simulink model "facedetection_demp"  (R2021b)
settings: Solver=FixedStepAuto  StartTime=0.0  StopTime=inf  RelTol=1e-3
undefined symbols (not defined in the file): Rec, SDTV
libraries: androiduilib x5, visionconversions x3, androidaudiovideolib x2, visiontextngfix x2, androidcommunicationlib x1
settings Model: Creator=The MathWorks, Inc.  LastModifiedBy=86150
settings SolverCC: AlgebraicLoopSolver=TrustRegion
settings DataIOCC: ReturnWorkspaceOutputs=off
settings OptimizationCC: EnhancedBackFolding=on  PassReuseOutputArgsThreshold=0  MaxStackSize=64  OptimizeBlockOrder=speed  DifferentSizesBufferReuse=on  OptimizationCustomize=off
settings DebuggingCC: ParameterTunabilityLossMsg=error  SFMachineParentedDataDiag=warning  ArithmeticOperatorsInVariantConditions=warning
settings HardwareCC: ProdBitPerPointer=32  ProdBitPerSizeT=32  ProdBitPerPtrDiffT=32  ProdLargestAtomicInteger=Long  ProdLargestAtomicFloat=Double  ProdWordSize=32  ProdHWDeviceType=ARM Compatible->ARM Cortex  UseEmbeddedCoderFeatures=off  UseSimulinkCoderFeatures=off
settings SFSimCC: CustomCodeUndefinedFunction=UseInterfaceOnly
settings RTWCC: Description=Embedded Coder  SystemTargetFile=ert.tlc  HardwareBoard=Android Device  TLCOptions="-aInlineSetEventsForThisBaseRateFcn=TLC_FALSE -aSuppressMultiTaskScheduler=TLC_FALSE  -aRateBasedStepFcn=0"  TemplateMakefile=ert_default_tmf  GenerateReport=on  RTWVerbose=off  Toolchain=Android SDK/NDK Tools  LaunchReport=on
settings CodeAppCC: ForceParamTrailComments=on  OperatorAnnotations=on
settings ERTTargetCC: ERTCustomFileBanners=off  SupportContinuousTime=on  SupportNonInlinedSFcns=on  RemoveResetFunc=off  SupportVariableSizeSignals=on  ModelStepFunctionPrototypeControlCompliant=off

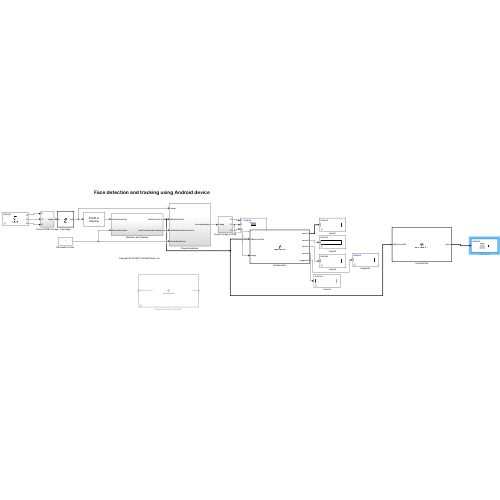
[thumbnail: Simulink's stored preview of the top-level diagram]
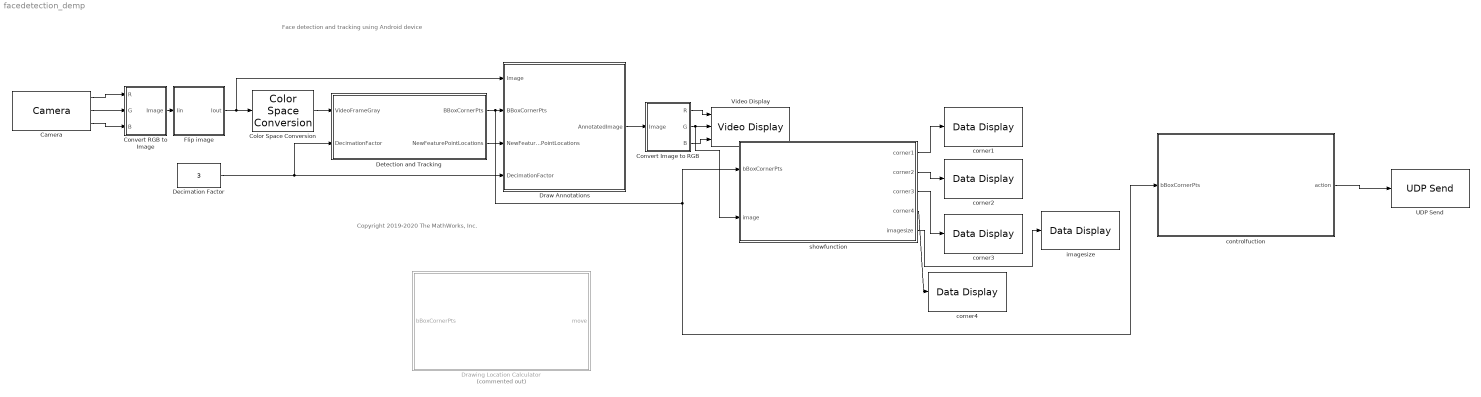
== system facedetection_demp ==
  note: Face detection and tracking using Android device
  note: Copyright 2019-2020 The MathWorks, Inc.
  Camera : androidaudiovideolib/Camera  CameraLocation=Back  CameraResolutions=Back - 640x480  Width=640  Height=480  SampleTime=0.1  BlockPlatform=Android
      settings: SourceProductBaseCode=ANDROID
  Color Space Conversion : visionconversions/Color Space  Conversion  conversion=Obsolete  conversionActive=R'G'B' to intensity  wp_str=D65  rec=Rec. 601 (SDTV)  sys=1125/60/2:1  imagePorts=One multidimensional signal
  Convert Image to RGB : Subsystem
  Convert RGB to Image : Subsystem
  Decimation Factor : Constant  Value=3
  Detection and Tracking : Subsystem
  Draw Annotations : Subsystem
  Drawing Location Calculator : MATLAB Function  Commented=on  TreatAsAtomicUnit=on
  Flip image : MATLAB Function  TreatAsAtomicUnit=on
  UDP Send : androidcommunicationlib/UDP Send  remoteURL='192.168.1.109'  remotePort=25000  localURL='0.0.0.0'  localPortSource=Automatically determine  localPort=-1  sampletime=-1  blockPlatform=Android  separateLengthPort=0
      settings: SourceProductBaseCode=ANDROID
  Video Display : androidaudiovideolib/Video Display  BlockPlatform=Android
      settings: SourceProductBaseCode=ANDROID
  controlfuction : MATLAB Function  TreatAsAtomicUnit=on
  corner1 : androiduilib/Data Display  DataDisplayId=facedetection_demp/corner1  Format=Float  Precision=6  SimulateUsing=Code generation  blockPlatform=Android
      settings: SourceProductBaseCode=ANDROID
  corner2 : androiduilib/Data Display  DataDisplayId=facedetection_demp/corner2  Format=Float  Precision=6  SimulateUsing=Code generation  blockPlatform=Android
      settings: SourceProductBaseCode=ANDROID
  corner3 : androiduilib/Data Display  DataDisplayId=facedetection_demp/corner3  Format=Float  Precision=6  SimulateUsing=Code generation  blockPlatform=Android
      settings: SourceProductBaseCode=ANDROID
  corner4 : androiduilib/Data Display  DataDisplayId=facedetection_demp/corner4  Format=Float  Precision=6  SimulateUsing=Code generation  blockPlatform=Android
      settings: SourceProductBaseCode=ANDROID
  imagesize : androiduilib/Data Display  DataDisplayId=facedetection_demp/imagesize  Format=Float  Precision=6  SimulateUsing=Code generation  blockPlatform=Android
      settings: SourceProductBaseCode=ANDROID
  showfunction : MATLAB Function  TreatAsAtomicUnit=on
  wires:
  Detection and Tracking/2(NewFeaturePointLocations) -> Draw Annotations/3(NewFeaturePointLocations)
  Detection and Tracking/1(BBoxCornerPts) -> controlfuction/1(bBoxCornerPts), showfunction/1(bBoxCornerPts), Draw Annotations/2(BBoxCornerPts)
  Color Space Conversion/1 -> Detection and Tracking/1(VideoFrameGray)
  Flip image/1(Iout) -> Draw Annotations/1(Image), Color Space Conversion/1
  Draw Annotations/1(AnnotatedImage) -> Convert Image to RGB/1(Image)
  Convert Image to RGB/1(R) -> Video Display/1
  Convert Image to RGB/2(G) -> showfunction/2(image), Video Display/2
  Convert Image to RGB/3(B) -> Video Display/3
  Convert RGB to Image/1(Image) -> Flip image/1(Iin)
  Camera/1 -> Convert RGB to Image/1(R)
  Camera/2 -> Convert RGB to Image/2(G)
  Camera/3 -> Convert RGB to Image/3(B)
  Decimation Factor/1 -> Draw Annotations/4(DecimationFactor), Detection and Tracking/2(DecimationFactor)
  showfunction/1(corner1) -> corner1/1
  showfunction/4(corner4) -> corner4/1
  showfunction/3(corner3) -> corner3/1
  showfunction/2(corner2) -> corner2/1
  showfunction/5(imagesize) -> imagesize/1
  controlfuction/1(action) -> UDP Send/1

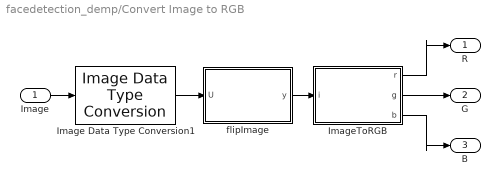
== system facedetection_demp/Convert Image to RGB ==
  Image : Inport
  Image Data Type Conversion1 : visionconversions/Image Data Type Conversion  outDT=uint8  isSigned=on  wordLen=16  numFracBits=0
      settings: SourceProductBaseCode=VP
  ImageToRGB : MATLAB Function  TreatAsAtomicUnit=on
  flipImage : MATLAB Function  TreatAsAtomicUnit=on
  R : Outport
  G : Outport  Port=2
  B : Outport  Port=3
  wires:
  ImageToRGB/3(b) -> B/1
  flipImage/1(y) -> ImageToRGB/1(i)
  Image Data Type Conversion1/1 -> flipImage/1(U)
  ImageToRGB/2(g) -> G/1
  ImageToRGB/1(r) -> R/1
  Image/1 -> Image Data Type Conversion1/1

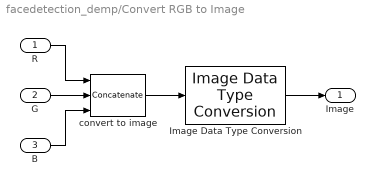
== system facedetection_demp/Convert RGB to Image ==
  R : Inport
  G : Inport  Port=2
  B : Inport  Port=3
  Image Data Type Conversion : visionconversions/Image Data Type Conversion  outDT=single  isSigned=on  wordLen=16  numFracBits=0
      settings: SourceProductBaseCode=VP
  convert to image : Concatenate  NumInputs=3  Mode=Multidimensional array  ConcatenateDimension=3
  Image : Outport
  wires:
  convert to image/1 -> Image Data Type Conversion/1
  B/1 -> convert to image/3
  G/1 -> convert to image/2
  R/1 -> convert to image/1
  Image Data Type Conversion/1 -> Image/1

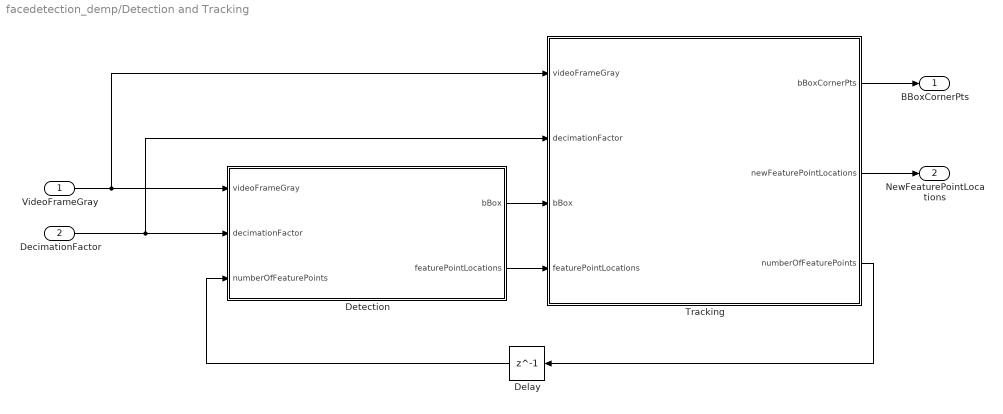
== system facedetection_demp/Detection and Tracking ==
  VideoFrameGray : Inport
  DecimationFactor : Inport  Port=2
  Delay : Delay  DelayLength=1
  Detection : MATLAB Function  TreatAsAtomicUnit=on
  Tracking : MATLAB Function  TreatAsAtomicUnit=on
  BBoxCornerPts : Outport  VectorParamsAs1DForOutWhenUnconnected=off
  NewFeaturePointLocations : Outport  Port=2  VectorParamsAs1DForOutWhenUnconnected=off
  wires:
  VideoFrameGray/1 -> Tracking/1(videoFrameGray), Detection/1(videoFrameGray)
  Detection/1(bBox) -> Tracking/3(bBox)
  Detection/2(featurePointLocations) -> Tracking/4(featurePointLocations)
  Tracking/1(bBoxCornerPts) -> BBoxCornerPts/1
  Tracking/2(newFeaturePointLocations) -> NewFeaturePointLocations/1
  DecimationFactor/1 -> Tracking/2(decimationFactor), Detection/2(decimationFactor)
  Tracking/3(numberOfFeaturePoints) -> Delay/1
  Delay/1 -> Detection/3(numberOfFeaturePoints)

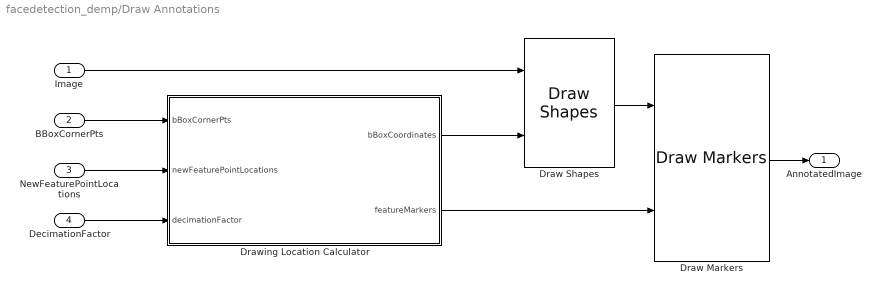
== system facedetection_demp/Draw Annotations ==
  Image : Inport
  BBoxCornerPts : Inport  Port=2
  NewFeaturePointLocations : Inport  Port=3
  DecimationFactor : Inport  Port=4
  Draw Markers : visiontextngfix/Draw Markers  shape=Plus  size=3  fill=off  fillClrSource=Specify via dialog  display=White  intensity=200  color=[200 255 100]  opacity=0.6  viewport=Entire image  antialiasing=off  inType=Obsolete  imagePorts=One multidimensional signal  roundingMode=Floor  overflowMode=off  memoryMode=Specify word length  memoryWordLength=16  memoryFracLength=15  prodOutputMode=Binary point scaling  prodOutputWordLength=32  prodOutputFracLength=14
      settings: SourceProductBaseCode=VP
  Draw Shapes : visiontextngfix/Draw Shapes  shape=Polygons  fill=off  lineWidth=1  fillClrSource=Specify via dialog  display=User-specified value  intensity=200  color=[255 255 0]  opacity=0.6  viewport=Entire image  antialiasing=off  inType=Obsolete  imagePorts=One multidimensional signal  roundingMode=Floor  overflowMode=off  memoryMode=Specify word length  memoryWordLength=16  prodOutputMode=Binary point scaling  prodOutputWordLength=32  prodOutputFracLength=14  memoryFracLength=14
  Drawing Location Calculator : MATLAB Function  TreatAsAtomicUnit=on
  AnnotatedImage : Outport  VectorParamsAs1DForOutWhenUnconnected=off
  wires:
  Drawing Location Calculator/1(bBoxCoordinates) -> Draw Shapes/2
  Draw Markers/1 -> AnnotatedImage/1
  Drawing Location Calculator/2(featureMarkers) -> Draw Markers/2
  Image/1 -> Draw Shapes/1
  BBoxCornerPts/1 -> Drawing Location Calculator/1(bBoxCornerPts)
  NewFeaturePointLocations/1 -> Drawing Location Calculator/2(newFeaturePointLocations)
  Draw Shapes/1 -> Draw Markers/1
  DecimationFactor/1 -> Drawing Location Calculator/3(decimationFactor)

== matlab function facedetection_demp/Detection and Tracking/Tracking ==
  data: videoFrameGray input; decimationFactor input; bBox input size=[2 8]; bBoxCornerPts output size=[4 2]; featurePointLocations input size=[500 2]; newFeaturePointLocations output size=[500 2]; numberOfFeaturePoints output
% Function for tracking face and feature points
%
% Copyright 2016 The MathWorks, Inc.
function [bBoxCornerPts, newFeaturePointLocations, numberOfFeaturePoints]  = trackPoints(videoFrameGray, decimationFactor, bBox, featurePointLocations)
%#codegen
persistent pointTracker
persistent oldPoints
persistent bboxPoints
persistent first_time
persistent numPts

% Create the point tracker object.
if isempty(pointTracker)
    pointTracker = vision.PointTracker('MaxBidirectionalError', 2);
end

if isempty(bboxPoints)
    bboxPoints = [0 0];
end 

if isempty(oldPoints)
    oldPoints = single([0 0]);
end      

if isempty(numPts)
    numPts = 0;
end

% Resize frame
videoFrameGray = videoFrameGray(1:decimationFactor:end,1:decimationFactor:end);

% Initialize tracker with dummy points
if isempty(first_time)
   initialize(pointTracker, single([10 10]), videoFrameGray);
   first_time = 0;
end

if numPts < 10
    if ~isempty(featurePointLocations)
        % Re-initialize the point tracker if a face has been detected and
        % feature points obtained.
        newFeaturePointLocations = featurePointLocations;
        numPts = size(newFeaturePointLocations,1);
        
        if ~pointTracker.isLocked
            initialize(pointTracker, newFeaturePointLocations, videoFrameGray);
        end
        step(pointTracker, videoFrameGray);
        setPoints(pointTracker, newFeaturePointLocations);
        
        % Save a copy of the points.
        oldPoints = newFeaturePointLocations;
        
        % Convert the rectangle represented as [x, y, w, h] into an
        % M-by-2 matrix of [x,y] coordinates of the four corners. This
        % is needed to be able to transform the bounding box to display
        % the orientation of the face.
        bboxPoints = bbox2points(bBox(1, :));
        bBoxCornerPts = bboxPoints;
    else
        bBoxCornerPts = [];
        newFeaturePointLocations = single([]);
    end

else
    % Tracking mode. 
    [newFeaturePointLocations, isFound] = step(pointTracker, videoFrameGray);
    assert(size(newFeaturePointLocations, 1) < 500);
    visiblePoints = newFeaturePointLocations(isFound, :);
    oldInliers = oldPoints(isFound, :);

    numPts = size(visiblePoints, 1);

    if numPts >= 10
        % Estimate the geometric transformation between the old points
        % and the new points.
        [xform, inlierIdx] = estimateGeometricTransform2D(...
            oldInliers, visiblePoints, 'similarity', 'MaxDistance', 4);
        visiblePoints = visiblePoints(inlierIdx, :);

        % Apply the transformation to the bounding box.
        bboxPoints = double(transformPointsForward(xform, bboxPoints));
        bBoxCornerPts = bboxPoints;

        % Assign the visible feature points
        assert(size(visiblePoints, 1) < 500);
        newFeaturePointLocations = visiblePoints;
        
        % Reset the points.
        oldPoints = visiblePoints;
        setPoints(pointTracker, oldPoints);
    else
        bBoxCornerPts = [];
        newFeaturePointLocations = single([]);            
    end

end

numberOfFeaturePoints = numPts;

== matlab function facedetection_demp/Detection and Tracking/Detection ==
  data: bBox output size=[2 8]; videoFrameGray input; featurePointLocations output size=[500 2]; decimationFactor input; numberOfFeaturePoints input
% Function for detecting a face and feature points.
%
% Copyright 2016 The MathWorks, Inc.
function [bBox, featurePointLocations]  = detectFaceAndFeatures(...
    videoFrameGray, decimationFactor, numberOfFeaturePoints)

%#codegen
persistent faceDetector

% Resize frame
videoFrameGray = videoFrameGray(1:decimationFactor:end,1:decimationFactor:end);

% Perform detection when the number of points being tracked goes below a
% certain threshold. These points may be just outliers.
%if numberOfFeaturePoints < 10
    % Detection mode
    
    % Create the face detector object.
    if isempty(faceDetector)
        faceDetector = vision.CascadeObjectDetector('/sdcard/haarcascade_frontalface_alt2.xml');
    end

    bBox = faceDetector.step(videoFrameGray);
    % Asser if a face is not detected.
    assert(size(bBox, 1) < 10);
    
    if ~isempty(bBox)
        % Find corner points inside the detected region.
        points = detectMinEigenFeatures(videoFrameGray, 'ROI', bBox(1, :));    
        featurePointLocations = points.Location;
    else
        % Return emtpty if no face detected.
        featurePointLocations = single([]);
    end
% else
%     % Return empty if once face is detected and valid.
%     bBox = [];
%     featurePointLocations = single([]);
% end

== matlab function facedetection_demp/Draw Annotations/Drawing Location Calculator ==
  data: bBoxCornerPts input size=[4 2]; bBoxCoordinates output size=[1 8]; newFeaturePointLocations input size=[500 2]; featureMarkers output size=[500 2]; decimationFactor input
% Function for calculating drawing locations
%
% Copyright 2016 The MathWorks, Inc.
function [bBoxCoordinates, featureMarkers]  = obtainDrawingLocations(bBoxCornerPts, newFeaturePointLocations, decimationFactor)

if ~isempty(bBoxCornerPts)
    % Convert the box corners into the [x1 y1 x2 y2 x3 y3 x4 y4]
    % format required by insertShape.
    bboxPolygon = reshape(bBoxCornerPts', 1, []);
    
    % Display a bounding box around the detected face.
    bBoxCoordinates = bboxPolygon.* decimationFactor;
   
    % Display detected corners.
    featureMarkers = newFeaturePointLocations.* decimationFactor;
else
    % Draw Markers and Draw Shapes block expect an input to be provided.
    % Hence providing the following input when nothing to be drawn.
    bBoxCoordinates = [0 0 0 0 0 0 0 0];
    featureMarkers = single([0 0]);
end

== matlab function facedetection_demp/Convert Image to RGB/ImageToRGB ==
  data: i input; r output; g output; b output
function [r, g, b] = ImageToRGB(i)
r=i(:,:,1);
g=i(:,:,2);
b=i(:,:,3);

== matlab function facedetection_demp/Flip image ==
  data: Iin input; Iout output
function Iout = flip(Iin)
%rotate image anti clockwise 90 degrees
Iin= imrotate( Iin , 90 );
%Flip image
Iin=flipdim(Iin,1);
Iout = Iin;

== matlab function facedetection_demp/Drawing Location Calculator ==
  data: bBoxCornerPts input size=[4 2]; move output size=[1 8]
% Function for calculating drawing locations
%
% Copyright 2016 The MathWorks, Inc.
function move   = movefuction(bBoxCornerPts)

if ~isempty(bBoxCornerPts)
    % Convert the box corners into the [x1 y1 x2 y2 x3 y3 x4 y4]
    % format required by insertShape.
    move = true;
    
    % Display a bounding box around the detected face.
else
    move = false;
end

== matlab function facedetection_demp/Convert Image to RGB/flipImage ==
  data: U input; y output
function y = flipImage(U)
U= imrotate( U , 90 );
%Flip image
U=flipdim(U,1);

y = U;

== matlab function facedetection_demp/showfunction ==
  data: bBoxCornerPts input size=[4 2]; corner1 output size=[1 8]; corner2 output; corner3 output; corner4 output; image input; imagesize output
% Function for calculating drawing locations
%
% Copyright 2016 The MathWorks, Inc.
function [corner1,corner2,corner3,corner4,imagesize]   = showfuction(bBoxCornerPts,image)

corner1 = bBoxCornerPts(1,1:2);
corner2 = bBoxCornerPts(2,1:2);
corner3 = bBoxCornerPts(3,1:2);
corner4 = bBoxCornerPts(4,1:2);
imagesize = size(image);

== matlab function facedetection_demp/controlfuction ==
  data: bBoxCornerPts input size=[4 2]; action output size=[1 8]
% Function for calculating drawing locations
%
% Copyright 2016 The MathWorks, Inc.
function action = controlfuction(bBoxCornerPts)


if isempty(bBoxCornerPts)
    action = 0;%停止
else
    corner1 = bBoxCornerPts(1,1:2);
    corner3 = bBoxCornerPts(3,1:2);
    x1 = (corner1+corner3)/2;
    x2 = [105 80];
    area = ((corner1(1)-corner3(1))^2+(corner1(2)-corner3(2))^2)/2;
    if area > 80*80
    action = 0;
    else 
        if x1(1)-x2(1)<-10
            action = 2;%左转
        elseif x1(1)-x2(1)>10
            action = 3;%右转
        else
            action = 1;%前进
        end        
    end
end
end
